simulink model "VCAL_APIS_A"  (R2023b)
settings: configuration reference "Configuration_Reference" (kept outside this file)
PreLoadFcn:
  | addpath('..\Common\');
  | Desktop_Configuration
InitFcn:
  | Desktop_Configuration
  | create_APIS_A_IO_bus();
undefined symbols (not defined in the file or in its folder): APIS_A_Status_enum
libraries: simulink x1
settings Model: Creator=IanM  LastModifiedBy=maxju
settings ConfigSetRef: SourceName=Configuration_Reference  SourceLocation=Base Workspace

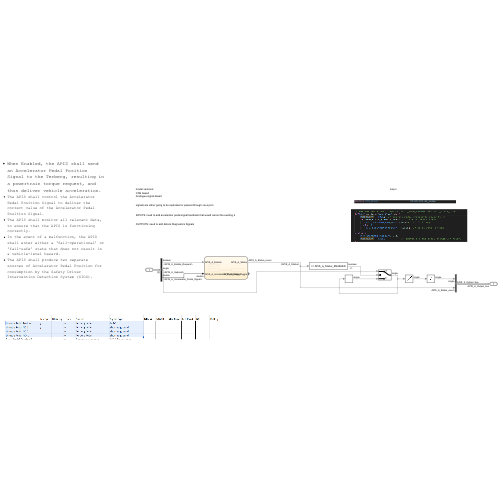
[thumbnail: Simulink's stored preview of the top-level diagram]
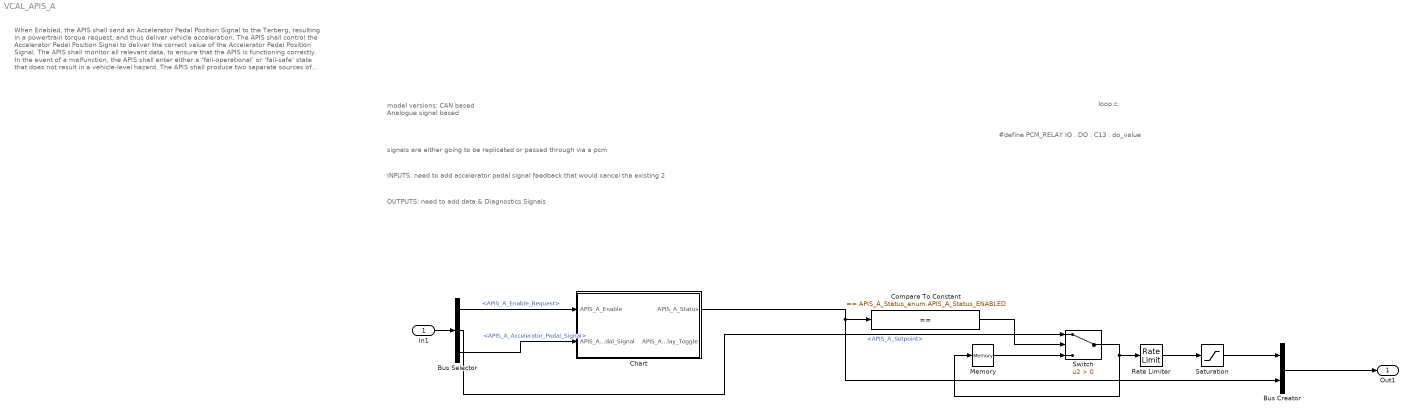
== system VCAL_APIS_A ==
  note: loop.c:
  note: #define PCM_RELAY IO . DO . C13 . do_value
  note: model versions:
      | CAN based
      | Analogue signal based
  note: signals are either going to be replicated or passed through via a pcm
  note: When Enabled, the APIS shall send an Accelerator Pedal Position Signal to the Terberg, resulting in a powertrain torque request, and thus deliver vehicle acceleration.
      | The APIS shall control the Accelerator Pedal Position Signal to deliver the correct value of the Accelerator Pedal Position Signal.
      | The APIS shall monitor all relevant data, to ensure that the APIS is functioning correctly.
      | In the event of a malfunction, the APIS shall enter either a ‘fail-operational’ or ‘fail-safe’ state that does not result in a vehicle-level hazard.
      | The APIS shall produce two separate sources of Accelerator Pedal Position for consumption by the Safety Driver Intervention Detection System (SIDS).
  note: OUTPUTS: need to add data & Diagnostics Signals
  note: INPUTS: need to add accelerator pedal signal feedback that would cancel the existing 2
  In1 : Inport  OutDataTypeStr=Bus: APIS_A_Input_bus
  Bus Creator : BusCreator  Inputs=2  OutDataTypeStr=Bus: APIS_A_Output_bus  NonVirtualBus=on
      settings: InheritFromInputs=off
  Bus Selector : BusSelector  OutputSignals=APIS_A_Enable_Request,APIS_A_Setpoint,APIS_A_Accelerator_Pedal_Signal
  Chart : Stateflow chart  TreatAsAtomicUnit=on
  Compare To Constant : simulink/Logic and Bit Operations/Compare To Constant  relop===  const=APIS_A_Status_enum.APIS_A_Status_ENABLED  OutDataTypeStr=boolean
  Memory : Memory
  Rate Limiter : RateLimiter  RisingSlewLimit=360  FallingSlewLimit=-360  SampleTimeMode=inherited
  Saturation : Saturate  UpperLimit=720  LowerLimit=-720
  Switch : Switch  Criteria=u2 > Threshold  SaturateOnIntegerOverflow=off  InputSameDT=off
  Out1 : Outport  OutDataTypeStr=Bus: APIS_A_Output_bus
  wires:
  In1/1 -> Bus Selector/1
  Bus Creator/1 -> Out1/1
  Bus Selector/2 -> Switch/1  "<APIS_A_Setpoint>"
  Rate Limiter/1 -> Saturation/1
  Chart/1(APIS_A_Status) -> Compare To Constant/1, Bus Creator/2
  Bus Selector/1 -> Chart/1(APIS_A_Enable)  "<APIS_A_Enable_Request>"
  Compare To Constant/1 -> Switch/2
  Saturation/1 -> Bus Creator/1
  Memory/1 -> Switch/3
  Switch/1 -> Rate Limiter/1, Memory/1
  Bus Selector/3 -> Chart/2(APIS_A_Accelerator_Pedal_Signal)  "<APIS_A_Accelerator_Pedal_Signal>"

== stateflow chart VCAL_APIS_A/Chart ==
  state Init
    APIS_A_Status = APIS_A_Status_enum.APIS_A_Status_INIT;
  state Disabled
    APIS_A_Status = APIS_A_Status_enum.APIS_A_Status_DISABLED;
  state Enabled
    APIS_A_Status = APIS_A_Status_enum.APIS_A_Status_ENABLED;
    APIS_A_Relay_Toggle = 1;
  (default) -> Init
  Init -> Disabled : after(1.0, sec)
  Disabled -> Enabled : [APIS_A_Accelerator_Pedal_Signal <1000 || APIS_A_Enable == true]
  Enabled -> Disabled : [APIS_A_Accelerator_Pedal_Signal >1000 || APIS_A_Enable == false]
  data: APIS_A_Enable input; APIS_A_Status output; APIS_A_Accelerator_Pedal_Signal input; APIS_A_Relay_Toggle output
